simulink model "rf_system_ofdm"  (R2022b)
settings: Solver=VariableStepAuto  StartTime=0.0  StopTime=10.0  RelTol=1e-3
PreLoadFcn:
  | clear;
  | 
  | % To extend frequency resolution down to lower frequencies,
  | % increase duration as well as the impulse response duration
  | % in the LO1 block mask
  | %clear;
  | rng(1000);
  | %load the minimum PAR sequence
  | load('DATA_SEQUENCES_256.mat');
  | tx_signal_ref = d_f_256(:,1:512);
  | 
  | 
  | % Number of Rx antennas (note: Since Tx beamforming is assumed for a single data stream, the receiver
  | % "sees" only a single transmit antenna); without loss of generarity, a ULA of N_rx elements is assumed for simplicity
  | N_rx = 24;
  | ovs = 8;
  | Num_Targets = 3;                    % Number of targets
  | range_distance = [80 250];          % range of values for distance
  | range_velocity = [-150 150];        % range of values for velocity (in km/h)
  | relative_power_range = [-20 0];     % range of relative power in dB (always set first target to 0 dB relative power)
  | azimuth_range = [75 105];           % in degrees (+/-15 degrees compared to boresight; 75 to 105 degrees from x-axis)
  | 
  | % generate range and velocity values per target (uniformly distributed)
  | Range = zeros(Num_Targets,1);
  | Velocity_kmh = zeros(Num_Targets,1);
  | Relative_power = zeros(Num_Targets,1);
  | for nn=1:Num_Targets
  |   Range(nn) = range_distance(1)+rand*(range_distance(2)-range_distance(1));
  |   Velocity_kmh(nn) = range_velocity(1)+rand*(range_velocity(2)-range_velocity(1));
  |   if nn > 1
  |       % set power only for targets 2:Num_Targets (first target is always at 0 dB relative power)
  |       Relative_power(nn) = relative_power_range(1)+rand*(relative_power_range(2)-relative_power_range(1));
  |   end
  |   Azimuth(nn) = azimuth_range(1)+rand*(azimuth_range(2)-azimuth_range(1));
  | end
  | % sort the distance values so that stronger targers appear with higher received power (as it usually happens in practice);
  | % accordingly, sort the velocity values
  | [Range, indices] = sort(Range,'ascend');
  | Velocity_kmh = Velocity_kmh(indices);
  | 
  | % general parameters
  | c0 = 3e08;
  | Fc = 77e09;
  | lambda = c0/Fc;
  | %SNR_dB = 100;           % relative to the target received with the lowest power!
  | 
  | % numerology
  | DF = 449.21875E03;
  | Nsc = 256;
  | T = 1/DF;
  | Ts = T/Nsc;
  | Tovs = Ts/ovs;    %added to account for oversampling H.M.
  | Ncp = 210;
  | Tcp = Ncp*Ts;
  | Tt = T+Tcp;
  | alpha_pri = 4;
  | Nsym = 512;
  | FrameDuration = Tt*alpha_pri*Nsym;
  | res_dist = c0/(2*Nsc*DF);                       % range resolution
  | res_vel = c0/(2*Fc*FrameDuration)*3.6;          % velocity resolution (in km/h)
  | 
  | % FFT/IFFT matrices
  | F_Nc = (1/sqrt(Nsc))*two_dim_matr_gen(1/Nsc/ovs,Nsc*ovs,Nsc*ovs);
  | %F_Nc = (1/sqrt(Nsc))*two_dim_matr_gen(1/Nsc,Nsc,Nsc);
  | iF_Nc = inv(F_Nc);
  | 
  | % range/Doppler windowing filters
  | tmpi = (1:Nsc).';
  | tmpf = 0.5*(1-cos(2*pi*tmpi/Nsc));
  | w_fast = diag( sqrt(1/real(tmpf'*tmpf))*tmpf );
  | tmpi = (1:Nsym).';
  | tmpf = 0.5*(1-cos(2*pi*tmpi/Nsym));
  | w_slow = diag( sqrt(Nsym/real(tmpf'*tmpf))*tmpf );
  | 
  | 
  | %interpolate using IFFT H.M.
  | 
  | z=zeros(Nsc*(ovs-1), Nsym);
  | hNsc = Nsc/2;
  | tsl= tx_signal_ref(1:hNsc,:);
  | tsh= tx_signal_ref(hNsc+1:Nsc,:);
  | tx_signal_ref_ovs=[tsl;z;tsh];
  | %output reference signal in time domain H.M.
  | td_tx_signal_ovs = iF_Nc*tx_signal_ref_ovs;   %time domain transmit signal
  | td_tx_signal_ovs = td_tx_signal_ovs(:);
  | %prepare to transfer data to simulink H.M.
  | time = Tovs*(0:length(td_tx_signal_ovs)-1);
  | time =time';
  | simin.time=time;
  | simin.signals.values=td_tx_signal_ovs;
  | 
  | 
  | carriers.LO = 22e9;
  | carriers.LOL = carriers.LO/2;
  | carriers.LOH = carriers.LO*3;
  | carriers.OUT = carriers.LO*3.5;
  | 
  | %Put all carriers in one vector for convenience
  | car_env = unique(structfun(@deal,carriers));
  | 
  | 
  | % Lower limit of frequency (governed by impulse duration):
  | Duration = Tovs*128;
  | LLFreq = 1/Duration;
  | 
  | 
  | %Upper limit of frequency (governed by sample time):
  | ULFreq = 1/(2*Tovs);
  | 
  | % Generate 1/f phase noise with -60dBc/Hz level @ 1KHz:
  | PhNoOffsets = [LLFreq 1e3 ULFreq];
  | PhNoLevels = -40-10*log10(PhNoOffsets/1e3);
libraries: simrfV2util1 x7, dspstat3 x5, simrfV2sources1 x2, simrfV2elements x1
settings Model: SimulationMode=accelerator  Creator=hessam  LastModifiedBy=hessam

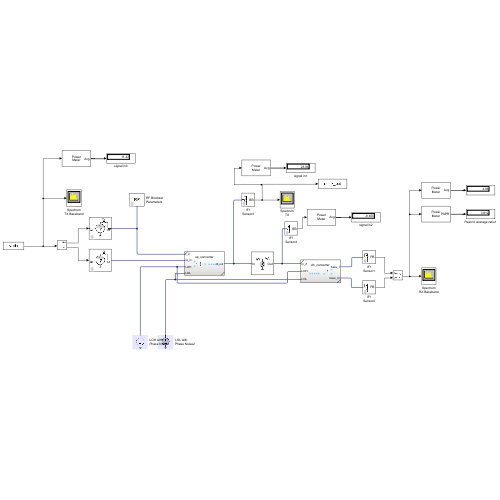
[thumbnail: Simulink's stored preview of the top-level diagram]
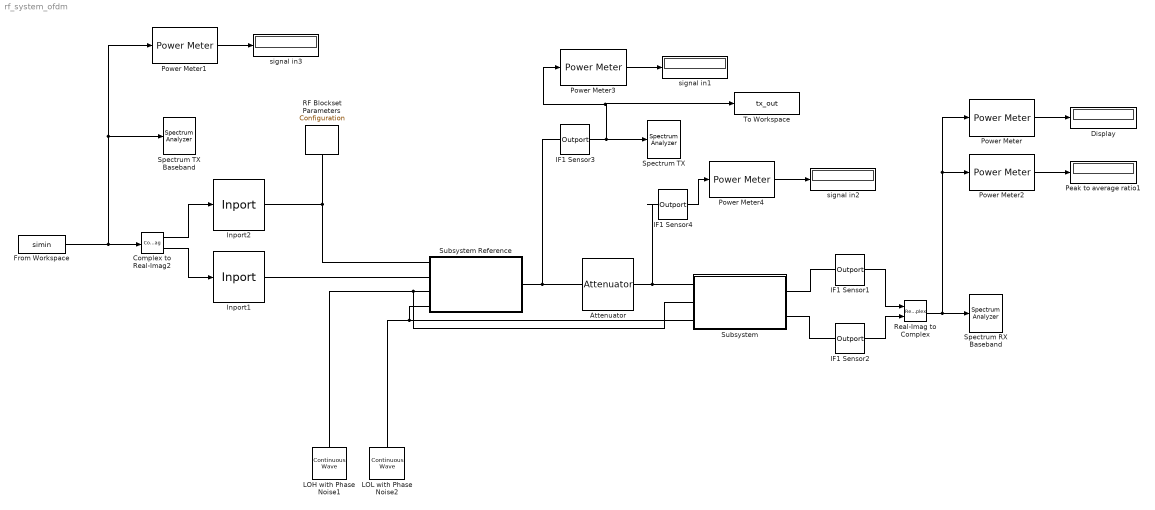
== system rf_system_ofdm ==
  Attenuator : simrfV2elements/Attenuator  classname=attenuator  Att=30  Zin=50  Zout=50  AddNoise=on  InternalGrounding=on
  Complex to Real-Imag2 : ComplexToRealImag
  Display : Display
  From Workspace : FromWorkspace  VariableName=simin  SampleTime=-1
  IF1 Sensor1 : simrfV2util1/Outport  SensorType=Power  OutputFormat=Real Passband  CarrierFreq=0 Hz  ZL=50  InternalGrounding=on  StepSize=-1 s  AutoStep=off
  IF1 Sensor2 : simrfV2util1/Outport  SensorType=Power  OutputFormat=Real Passband  CarrierFreq=0 Hz  ZL=50  InternalGrounding=on  StepSize=-1 s  AutoStep=off
  IF1 Sensor3 : simrfV2util1/Outport  SensorType=Power  OutputFormat=Complex Baseband  CarrierFreq=carriers.OUT Hz  ZL=50  InternalGrounding=on  StepSize=-1 s  AutoStep=off
  IF1 Sensor4 : simrfV2util1/Outport  SensorType=Power  OutputFormat=Complex Baseband  CarrierFreq=carriers.OUT Hz  ZL=50  InternalGrounding=on  StepSize=-1 s  AutoStep=off
  Inport1 : simrfV2util1/Inport  SimulinkInputSignalType=Power  CarrierFreq=0 Hz  ZS=50  UseSqWave=off  NumCoeff=10  Bias=0  DutyCyc=50  InternalGrounding=on
  Inport2 : simrfV2util1/Inport  SimulinkInputSignalType=Power  CarrierFreq=0 Hz  ZS=50  UseSqWave=off  NumCoeff=10  Bias=0  DutyCyc=50  InternalGrounding=on
  LOH with Phase Noise1 : simrfV2sources1/Continuous Wave  CWSourceType=Ideal voltage  Z0=0  IVoltage=1 V  ICurrent=0 A  MagPower=0 W  QVoltage=0 V  QCurrent=0 A  AnglePower=0  CarrierFreq=carriers.LOH Hz  AddPhaseNoise=off  PhaseNoiseOffset=PhNoOffsets  PhaseNoiseLevel=PhNoLevels  AutoImpulseLength=on  ImpulseLength=1e-10 s  InternalGrounding=on
  LOL with Phase Noise2 : simrfV2sources1/Continuous Wave  CWSourceType=Ideal voltage  Z0=0  IVoltage=1 V  ICurrent=0 A  MagPower=0 W  QVoltage=0 V  QCurrent=0 A  AnglePower=0  CarrierFreq=carriers.LOL Hz  AddPhaseNoise=on  PhaseNoiseOffset=PhNoOffsets  PhaseNoiseLevel=PhNoLevels  AutoImpulseLength=on  ImpulseLength=1e-10 s  InternalGrounding=on
  Peak to average ratio1 : Display
  Power Meter : dspstat3/Power Meter  Measurement=Average power  ReferenceLoad=1  OutputPowerUnits=dBm  WindowLength=1024  OverlapLength=1023  AllowArbitraryInputLength=on  ComputeCCDF=off  PowerRange=50  PowerResolution=0.1  CCDFOutput=Relative power (dB above average power)  ProbabilityVector=[ 10; 1; 0.1; 0.01; 0.001; 0.0001 ]  RelativePowerVector=[ 0; 3; 6; 9; 12 ]  ResetPort=off  SimulateUsing=Code generation
      settings: LibrarySourceBlock=commutil2/Power Meter
  Power Meter1 : dspstat3/Power Meter  Measurement=Average power  ReferenceLoad=1  OutputPowerUnits=dBm  WindowLength=256  OverlapLength=255  AllowArbitraryInputLength=on  ComputeCCDF=off  PowerRange=50  PowerResolution=0.1  CCDFOutput=Relative power (dB above average power)  ProbabilityVector=[ 10; 1; 0.1; 0.01; 0.001; 0.0001 ]  RelativePowerVector=[ 0; 3; 6; 9; 12 ]  ResetPort=off  SimulateUsing=Code generation
      settings: LibrarySourceBlock=commutil2/Power Meter
  Power Meter2 : dspstat3/Power Meter  Measurement=Peak-to-average power ratio  ReferenceLoad=1  OutputPowerUnits=dBm  WindowLength=256  OverlapLength=255  AllowArbitraryInputLength=on  ComputeCCDF=off  PowerRange=50  PowerResolution=0.1  CCDFOutput=Relative power (dB above average power)  ProbabilityVector=[ 10; 1; 0.1; 0.01; 0.001; 0.0001 ]  RelativePowerVector=[ 0; 3; 6; 9; 12 ]  ResetPort=off  SimulateUsing=Code generation
      settings: LibrarySourceBlock=commutil2/Power Meter
  Power Meter3 : dspstat3/Power Meter  Measurement=Average power  ReferenceLoad=1  OutputPowerUnits=dBm  WindowLength=256  OverlapLength=255  AllowArbitraryInputLength=on  ComputeCCDF=off  PowerRange=50  PowerResolution=0.1  CCDFOutput=Relative power (dB above average power)  ProbabilityVector=[ 10; 1; 0.1; 0.01; 0.001; 0.0001 ]  RelativePowerVector=[ 0; 3; 6; 9; 12 ]  ResetPort=off  SimulateUsing=Code generation
      settings: LibrarySourceBlock=commutil2/Power Meter
  Power Meter4 : dspstat3/Power Meter  Measurement=Average power  ReferenceLoad=1  OutputPowerUnits=dBm  WindowLength=256  OverlapLength=255  AllowArbitraryInputLength=on  ComputeCCDF=off  PowerRange=50  PowerResolution=0.1  CCDFOutput=Relative power (dB above average power)  ProbabilityVector=[ 10; 1; 0.1; 0.01; 0.001; 0.0001 ]  RelativePowerVector=[ 0; 3; 6; 9; 12 ]  ResetPort=off  SimulateUsing=Code generation
      settings: LibrarySourceBlock=commutil2/Power Meter
  RF Blockset Parameters : simrfV2util1/Configuration  AutoFreq=on  Tones="[11  66] GHz"  Harmonics="[5  5]"  NormalizeCarrierPower=on  SolverType=Auto  UseCCode=on  StepSize=Tovs s  AddNoise=off  defaultRNG=on  Seed=0  Temperature=293.15 K  SolverDelFlag=0  AbsTol=1e-6  RelTol=1e-3  MaxIter=10  ErrorEstimationType=2-norm over all variables  EnableInterpFilter=off  HiddenFIRfilterControllerParam=off  SmallSignalApprox=off  AllSimFreqs=on  SimFreqs=[] Hz  SimFreqsInternal=[]  SamplesPerFrame=1
  Real-Imag to Complex : RealImagToComplex
  Spectrum RX Baseband : SpectrumAnalyzer
  Spectrum TX : SpectrumAnalyzer
  Spectrum TX Baseband : SpectrumAnalyzer
  Subsystem : Subsystem  ReferencedSubsystem=dn_converter
      settings: PortSchema="{\"entries\":[{\"content\":{\"sides\":[{\"content\":{\"connectorIds\":[\"LConn3\",\"LConn1\",\"LConn2\"]},\"type\":\"ConnectorPlacement.EquallySpacedRectSide\",\"uuid\":\"8336b51e-e5d8-49cc-804f-7bfb99400ab0\"},{\"content\":{\"connectorIds\":[\"LConn4\",\"LConn5\"],\"side\":\"RIGHT\"},\"type\":\"ConnectorPlacement.EquallySpacedRectSide\",\"uuid\":\"6f005c77-3014-47d2-89f9-41814728faba\"},{\"content\":{\"connectorIds\":[],\"side\":\"TOP\"},\"type\":\"ConnectorPlacement.EquallySpacedRectSide\",\"uuid\":\"edcdef5b-1b73-4458-84fc-72d761e40cdf\"}]},\"type\":\"ConnectorPlacement.EquallySpacedConnector\",\"uuid\":\"3f0b5c66-2f3f-40e5-bb1c-488293219f70\"}],\"packageUris\":[\"http://schema.mathworks.com/mf0/Connector/R2020b\"],\"version\":\"1.0\"}"
  Subsystem Reference : Subsystem  ReferencedSubsystem=up_converter
      settings: PortSchema="{\"entries\":[{\"content\":{\"sides\":[{\"content\":{\"connectorIds\":[\"LConn3\",\"LConn4\",\"LConn2\",\"LConn1\"]},\"type\":\"ConnectorPlacement.EquallySpacedRectSide\",\"uuid\":\"8336b51e-e5d8-49cc-804f-7bfb99400ab0\"},{\"content\":{\"connectorIds\":[\"LConn5\"],\"side\":\"RIGHT\"},\"type\":\"ConnectorPlacement.EquallySpacedRectSide\",\"uuid\":\"6f005c77-3014-47d2-89f9-41814728faba\"},{\"content\":{\"connectorIds\":[],\"side\":\"TOP\"},\"type\":\"ConnectorPlacement.EquallySpacedRectSide\",\"uuid\":\"edcdef5b-1b73-4458-84fc-72d761e40cdf\"}]},\"type\":\"ConnectorPlacement.EquallySpacedConnector\",\"uuid\":\"3f0b5c66-2f3f-40e5-bb1c-488293219f70\"}],\"packageUris\":[\"http://schema.mathworks.com/mf0/Connector/R2020b\"],\"version\":\"1.0\"}"
  To Workspace : ToWorkspace  VariableName=tx_out  SampleTime=-1
  signal in1 : Display
  signal in2 : Display
  signal in3 : Display
  wires:
  Complex to Real-Imag2/1 -> Inport2/1
  Complex to Real-Imag2/2 -> Inport1/1
  IF1 Sensor1/1 -> Real-Imag to Complex/1
  Power Meter/1 -> Display/1
  Real-Imag to Complex/1 -> Power Meter2/1, Power Meter/1, Spectrum RX Baseband/1
  Power Meter2/1 -> Peak to average ratio1/1
  IF1 Sensor2/1 -> Real-Imag to Complex/2
  IF1 Sensor3/1 -> To Workspace/1, Power Meter3/1, Spectrum TX/1
  Power Meter3/1 -> signal in1/1
  Power Meter4/1 -> signal in2/1
  IF1 Sensor4/1 -> Power Meter4/1
  From Workspace/1 -> Power Meter1/1, Spectrum TX Baseband/1, Complex to Real-Imag2/1
  Power Meter1/1 -> signal in3/1
  connections:
  Subsystem Reference/LConn5 -- IF1 Sensor3/LConn1 -- Attenuator/LConn1
  Subsystem/LConn3 -- IF1 Sensor4/LConn1 -- Attenuator/RConn1
  Subsystem/LConn1 -- LOH with Phase Noise1/LConn1 -- Subsystem Reference/LConn2
  LOL with Phase Noise2/LConn1 -- Subsystem/LConn2 -- Subsystem Reference/LConn1
  RF Blockset Parameters/LConn1 -- Subsystem Reference/LConn3 -- Inport2/RConn1
  Subsystem Reference/LConn4 -- Inport1/RConn1
  Subsystem/LConn5 -- IF1 Sensor2/LConn1
  Subsystem/LConn4 -- IF1 Sensor1/LConn1
